simulink model "TestLogPressione"  (R2013a)
settings: Solver=FixedStepDiscrete  StartTime=0.0  StopTime=inf  FixedStep=0.02  RelTol=1e-3
undefined symbols (not defined in the file or in its folder): serial
libraries: etargetslib x2, instrumentlib x2
settings Model: Creator=mine  LastModifiedBy=BCI-USER

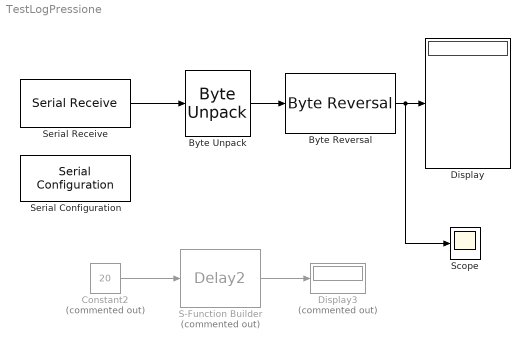
== system TestLogPressione ==
  Byte Reversal : etargetslib/Byte Reversal  numInp=1
  Byte Unpack : etargetslib/Byte Unpack  dimensions={[1]}  datatypes={'int32'}  byteAlign=1
  Constant2 : Constant  Commented=on  Value=20  OutDataTypeStr=uint32  SampleTime=-1
  Display : Display
  Display3 : Display  Commented=on
  S-Function Builder : S-Function  Commented=on  InitFcn=try, set_param(gcb,'FunctionName','Delay2'), end  FunctionName=Delay2  SFunctionModules=Delay2_wrapper  EnableBusSupport=off  mask(S-Function Builder){}
      mask help: Simulink:masks:SFunctionBuilder_MD
      mask init:
      | val = [[.9  0.75 0.75 1 1 .9 .9 1]',[1 1 0.75 0.75 .9 .9 1 .9]'];try , sys = get_param(gcb,'SfunBuilderFcnName');if isempty(sys), sys = get_param(gcb,'FunctionName'); end,catch, sys = get_param(gcb,'FunctionName'); end
      settings: CopyFcn=set_param(gcbh,'LinkStatus','none')  PreSaveFcn=try, set_param(gcb,'FunctionName','Delay2'), end  OpenFcn=sfunctionwizard(gcbh)
      mask Display: plot(val(:,1),val(:,2)),disp(sys), port_label('input',1,'u0'), port_label('output',1,'y0')
  Scope : Scope
      settings: YMin=237000  YMax=244500
  Serial Configuration : instrumentlib/Serial Configuration  Priority=-200000  ComPortMenu=COM23  ComPort=COM23  ObjConstructor=serial('COM23');  BaudRate=115200  DataBits=8  Parity=none  StopBits=1  FlowControl=none  Timeout=5  ByteOrder=LittleEndian
  Serial Receive : instrumentlib/Serial Receive  ComPortMenu=COM23  ComPort=COM23  ObjConstructor=serial('COM23');  Terminator=<none>  DataSize="[4  1]"  DataType=uint8  EnableBlockingMode=on  ActionDataUnavailable=Output last received value  CustomValue=0  SampleTime=-1
  wires:
  Constant2/1 -> S-Function Builder/1
  S-Function Builder/1 -> Display3/1
  Serial Receive/1 -> Byte Unpack/1
  Byte Reversal/1 -> Scope/1, Display/1
  Byte Unpack/1 -> Byte Reversal/1
